simulink model "CessnaLmdl"  (R2017b)
settings: Solver=VariableStepAuto  StartTime=0.0  StopTime=simtime  RelTol=1e-3
values from neighbouring files (symbols this model uses):
  x0 = [V0;alpha0;theta0;q0;0]    [Cessna_Simulation.m]
undefined symbols (not defined in the file or in its folder): A, B, C, D, x
settings Model: Creator=stroll  LastModifiedBy=stroll

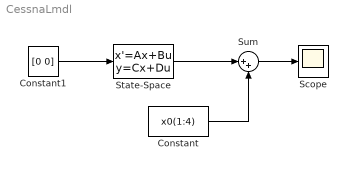
== system CessnaLmdl ==
  Constant : Constant  Value=x0(1:4)
  Constant1 : Constant  Value=[0 0]
  Scope : Scope
  State-Space : StateSpace  A=A  B=B  C=C  D=D  InitialCondition=x0(1:4) - x(1:4) + [5;0;0;0]
  Sum : Sum  Inputs=|++
  wires:
  State-Space/1 -> Sum/1
  Constant/1 -> Sum/2
  Sum/1 -> Scope/1
  Constant1/1 -> State-Space/1
